simulink model "task41"  (R2015b)
settings: Solver=VariableStepAuto  StartTime=0.0  StopTime=10.0  RelTol=1e-3
settings Model: Creator=Martin  LastModifiedBy=Martin

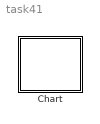
== system task41 ==
  Chart : Stateflow chart  TreatAsAtomicUnit=on

== stateflow chart task41/Chart ==
  state M2
    state Idle
    state Processing
    state Down
    (default) -> M2.Idle [order 1]
    (default) -> M2.Idle [order 4] : Repair
    (default) -> M2.Processing [order 2] : Start
    (default) -> M2.Idle [order 3] : End
    M2.Processing -> M2.Down : Breakdown
  state M1
    state Idle
    state Processing
    state Down
    (default) -> M1.Idle [order 1]
    (default) -> M1.Idle [order 4] : Repair
    (default) -> M1.Processing [order 2] : Start
    (default) -> M1.Idle [order 3] : End
    M1.Processing -> M1.Down : Breakdown
  state Buffer
    state Empty
    state Full
    (default) -> Empty [order 2]
    Full -> Empty : Taken
    (default) -> Full [order 1] : Placed
